simulink model "observador"  (R2021a)
settings: Solver=VariableStepAuto  StartTime=0.0  StopTime=10  RelTol=1e-3
settings Model: Creator=Jorge_Sarmiento  LastModifiedBy=Jorge_Sarmiento

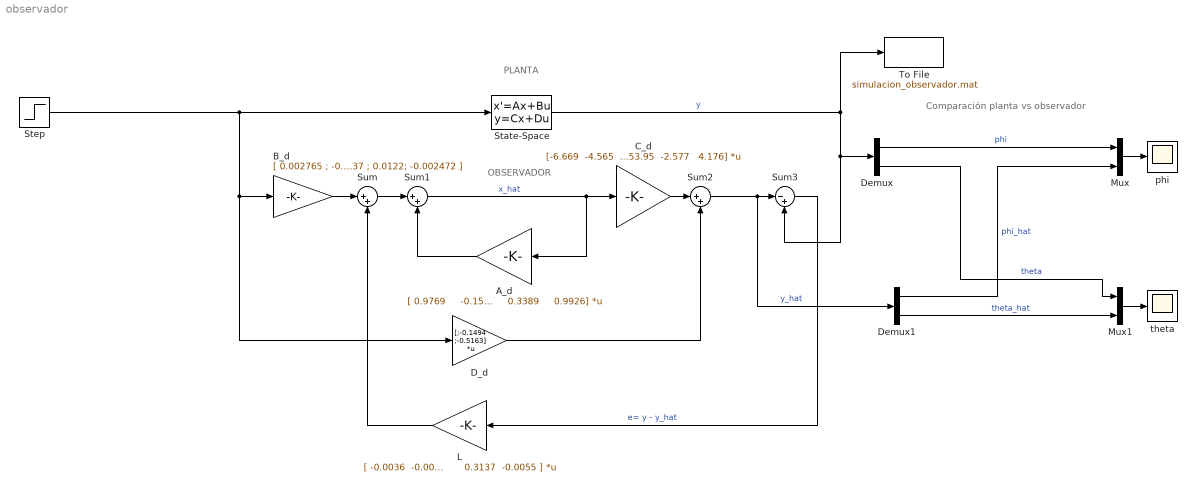
== system observador ==
  note: PLANTA
  note: OBSERVADOR
  note: Comparación planta vs observador
  A_d : Gain  Gain="[ 0.9769     -0.152  -0.001215   -0.02181;   0.1523     0.9838   -0.02593   0.008431;   -0.02706   -0.05485        0.8    -0.0522;   0.004625    0.03261     0.3389     0.9926]"  Multiplication=Matrix(K*u)
  B_d : Gain  Gain=|
      | [ 0.002765
      | ; -0.00137
      | ; 0.0122; -0.002472
      | ]
  C_d : Gain  Gain="[-6.669  -4.565  -19.02   6.812; -341.3   53.95  -2.577   4.176]"  Multiplication=Matrix(K*u)
  D_d : Gain  Gain=|  Multiplication=Matrix(K*u)
      | [;-0.1494
      | ;-0.5163]
  Demux : Demux  Outputs=2
  Demux1 : Demux  Outputs=2
  L : Gain  Gain=|  Multiplication=Matrix(K*u)
      | [ -0.0036  -0.0027;
      |       -0.0412   0.0159;
      |        0.0391  -0.0049;
      |        0.3137  -0.0055 ]
  Mux : Mux  Inputs=2
  Mux1 : Mux  Inputs=2
  State-Space : StateSpace  A=|  B="[0.1323;  -0.06944;  0.6708;   -0.23731]"  C="[-6.619   -5.83  -22.39   6.203;  -347.5   27.68  -2.737  0.2003]"  D=[0; 0]  InitialCondition=0  ParameterTunability=Unconstrained
      | [  -0.5739    -7.69  0.02236   -1.068;    7.703  -0.2749   -1.527   0.4686;  -1.268   -3.108   -10.61   -2.898
      | ;    0.323    2.188    18.84   0.1148]
  Step : Step  Time=0.1  After=20  SampleTime=0.02
  Sum : Sum  Inputs=|++
  Sum1 : Sum  Inputs=|++
  Sum2 : Sum  Inputs=|++
  Sum3 : Sum  Inputs=|-+
  To File : ToFile  Filename=simulacion_observador.mat  MatrixName=simulacion_observador  SaveFormat=Timeseries
  phi : Scope
  theta : Scope
  wires:
  State-Space/1 -> To File/1, Demux/1, Sum3/2  "y"
  B_d/1 -> Sum/1
  Sum/1 -> Sum1/1
  A_d/1 -> Sum1/2
  Sum1/1 -> A_d/1, C_d/1  "x_hat"
  C_d/1 -> Sum2/1
  Step/1 -> State-Space/1, D_d/1, B_d/1
  D_d/1 -> Sum2/2
  Sum2/1 -> Demux1/1, Sum3/1  "y_hat"
  Sum3/1 -> L/1  "e= y - y_hat"
  L/1 -> Sum/2
  Mux/1 -> phi/1
  Mux1/1 -> theta/1
  Demux/1 -> Mux/1  "phi"
  Demux1/1 -> Mux/2  "phi_hat"
  Demux/2 -> Mux1/1  "theta"
  Demux1/2 -> Mux1/2  "theta_hat"
